simulink model "lab"  (R2018a)
settings: Solver=VariableStepAuto  StartTime=0.0  StopTime=10.0  RelTol=1e-3
libraries: dsparch4 x1
settings Model: Creator=salman  LastModifiedBy=salman

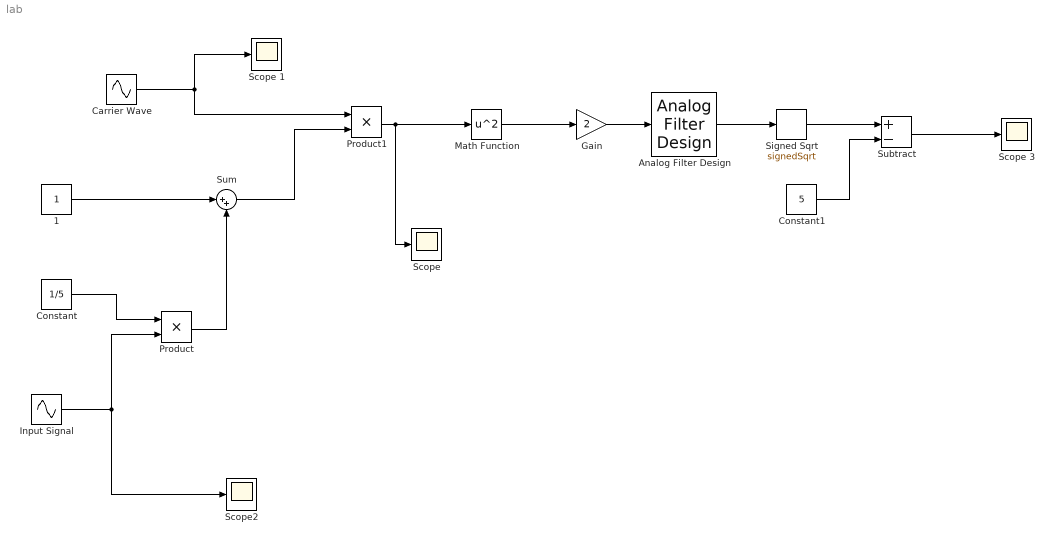
== system lab ==
  "1 " : Constant
  Analog Filter Design : dsparch4/Analog Filter Design  method=Butterworth  filttype=Lowpass  N=8  Wlo=30  Whi=80  Rp=2  Rs=40
  "Carrier Wave " : Sin  Amplitude=5  Frequency=2*pi*25  SampleTime=1/8000
  Constant : Constant  Value=1/5
  Constant1 : Constant  Value=5
  Gain : Gain  Gain=2
  Input Signal : Sin  Frequency=2*pi  SampleTime=1/8000
  Math Function : Math  Operator=square  SaturateOnIntegerOverflow=on
  Product : Product
  Product1 : Product
  "Scope " : Scope
  Scope 1 : Scope
  Scope 3 : Scope
  Scope2 : Scope
  Signed Sqrt : Sqrt  Operator=signedSqrt  SaturateOnIntegerOverflow=on
  Subtract : Sum  Inputs=+-
  Sum : Sum  Inputs=|++
  wires:
  Constant/1 -> Product/1
  "1 "/1 -> Sum/1
  Product/1 -> Sum/2
  "Carrier Wave "/1 -> Product1/1, Scope 1/1
  Sum/1 -> Product1/2
  Product1/1 -> Math Function/1, "Scope "/1
  Math Function/1 -> Gain/1
  Gain/1 -> Analog Filter Design/1
  Analog Filter Design/1 -> Signed Sqrt/1
  Signed Sqrt/1 -> Subtract/1
  Constant1/1 -> Subtract/2
  Subtract/1 -> Scope 3/1
  Input Signal/1 -> Scope2/1, Product/2
